simulink model "mpc_cvxgen_test"  (R2015b)
settings: Solver=VariableStepAuto  StartTime=0.0  StopTime=50  RelTol=1e-3
settings Model: Creator=Daniel  LastModifiedBy=mgreiff
settings SolverCC: AlgebraicLoopSolver=LineSearch

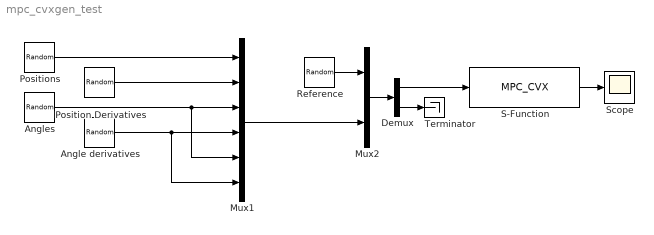
== system mpc_cvxgen_test ==
  Angle derivatives : RandomNumber  Variance=0.1  SampleTime=0.1
  Angles : RandomNumber  Variance=0.1  SampleTime=0.1
  Demux : Demux  Outputs=[10,3]
  Mux1 : Mux  Inputs=6
  Mux2 : Mux  Inputs=2
  Position Derivatives : RandomNumber  Mean=[0,0,0]  Variance=0.1  SampleTime=0.1
  Positions : RandomNumber  Mean=[0,0,0]  Variance=0.1  SampleTime=0.1
  Reference : RandomNumber  Mean=[0,0,0]  Variance=0.1  SampleTime=0.1
  S-Function : S-Function  FunctionName=MPC_CVX  Parameters=CVXparameters  SFunctionDeploymentMode=off  EnableBusSupport=off
  Scope : Scope
  Terminator : Terminator
  wires:
  Angles/1 -> Mux1/5, Mux1/3
  Angle derivatives/1 -> Mux1/6, Mux1/4
  Positions/1 -> Mux1/1
  Position Derivatives/1 -> Mux1/2
  S-Function/1 -> Scope/1
  Mux1/1 -> Mux2/2
  Reference/1 -> Mux2/1
  Demux/2 -> Terminator/1
  Mux2/1 -> Demux/1
  Demux/1 -> S-Function/1
